simulink model "soc_swhw_fpga"  (R2021a)
settings: Solver=VariableStepAuto  StartTime=0.0  StopTime=stopTime  RelTol=1e-3  EnableMultiTasking=on
PreLoadFcn:
  | hsb.blkcb2.defineTypes;
undefined symbols (not defined in the file): a, b, Bias1, Bias2, c, frameSize, jsin, LUT_Z0, LUT_Z1, NumBits1, NumBits2, quantizationBits, sampleTime, SF, Slope1, Slope2
libraries: simulink x42, hdlsllib x24, embreciprocals x4, hwlogicconnlib x4, dsphdlxfrm x2, dsphdlmathfun x1
(part 1 of 2)
settings Model: Creator=The MathWorks, Inc.  LastModifiedBy=AliReza
settings SolverCC: AlgebraicLoopSolver=TrustRegion  PositivePriorityOrder=on
settings DataIOCC: ReturnWorkspaceOutputs=off
settings OptimizationCC: DefaultParameterBehavior=Inlined  EnhancedBackFolding=on  PassReuseOutputArgsAs=Individual arguments  MaxStackSize=64  OptimizeBlockOrder=speed  DifferentSizesBufferReuse=on  OptimizationCustomize=off  EfficientTunableParamExpr=on
settings DebuggingCC: SignalRangeChecking=warning  ParameterTunabilityLossMsg=error  SFMachineParentedDataDiag=warning  ArithmeticOperatorsInVariantConditions=warning
settings HardwareCC: ProdBitPerPointer=32  ProdBitPerSizeT=32  ProdBitPerPtrDiffT=32  ProdLargestAtomicFloat=None  ProdIntDivRoundTo=Undefined  ProdEndianess=Unspecified  ProdWordSize=32  ProdHWDeviceType=ASIC/FPGA->ASIC/FPGA  TargetBitPerPointer=64  TargetBitPerSizeT=64  TargetBitPerPtrDiffT=64  TargetLongLongMode=on  TargetIntDivRoundTo=Zero  TargetEndianess=LittleEndian  TargetWordSize=64  TargetHWDeviceType=Custom Processor->MATLAB Host Computer  ProdEqTarget=off
settings SFSimCC: SimUseLocalCustomCode=off  MATLABDynamicMemAlloc=off
settings RTWCC: SystemTargetFile=ert.tlc  TemplateMakefile=ert_default_tmf  GenerateReport=on  RTWUseLocalCustomCode=off  Toolchain=Linaro AArch32 Linux v6.3.1  IncludeHyperlinkInReport=on  LaunchReport=on  GenerateTraceInfo=on  GenerateTraceReport=on  GenerateTraceReportSl=on  GenerateTraceReportSf=on  GenerateTraceReportEml=on
settings CodeAppCC: ForceParamTrailComments=on  IgnoreCustomStorageClasses=off  OperatorAnnotations=on  SimulinkDataObjDesc=on  SFDataObjDesc=on  InsertBlockDesc=on
settings ERTTargetCC: ERTCustomFileTemplate=example_file_process.tlc

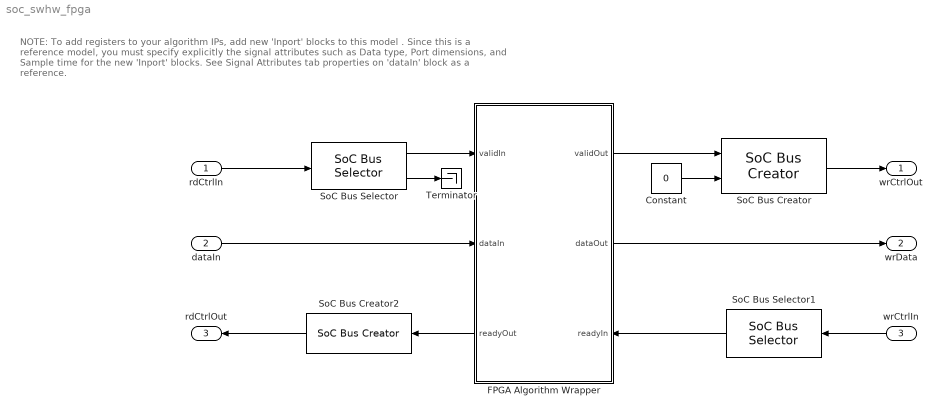
== system soc_swhw_fpga ==
  note: NOTE:
      | To add registers to your algorithm IPs, add new 'Inport' blocks to this model . Since this is a reference model, you must specify explicitly the signal attributes such as Data type, Port dimensions, and Sample time for the new 'Inport' blocks. See Signal Attributes tab properties on 'dataIn' block as a reference.
  rdCtrlIn : Inport  OutDataTypeStr=Bus: StreamM2SBusObj  SampleTime=sampleTime
  dataIn : Inport  Port=2  OutDataTypeStr=fixdt(1,32,30)  SampleTime=sampleTime
  wrCtrlIn : Inport  Port=3  OutDataTypeStr=Bus: StreamS2MBusObj  SampleTime=sampleTime
  Constant : Constant  Value=0  OutDataTypeStr=boolean  SampleTime=sampleTime
  FPGA Algorithm Wrapper : Subsystem  TreatAsAtomicUnit=on
      settings: PortSchema="{\"entries\":[{\"content\":{\"sides\":[{\"content\":{\"connectorIds\":[\"In1\",\"In2\",\"Out3\"]},\"type\":\"ConnectorPlacement.EquallySpacedRectSide\",\"uuid\":\"ebbc010d-f6ed-4988-870b-259581305fe2\"},{\"content\":{\"connectorIds\":[\"Out1\",\"Out2\",\"In3\"],\"side\":\"RIGHT\"},\"type\":\"ConnectorPlacement.EquallySpacedRectSide\",\"uuid\":\"4c5f59b6-7994-4c6f-b220-a18d8cf0d52f\"},{\"content\":{\"connectorIds\":[],\"side\":\"TOP\"},\"type\":\"ConnectorPlacement.EquallySpacedRectSide\",\"uuid\":\"7f6aff54-293a-4a30-be7c-233675f72493\"}]},\"type\":\"ConnectorPlacement.EquallySpacedConnector\",\"uuid\":\"db962109-073c-4896-87dc-fdd91b0482ef\"}],\"packageUris\":[\"http://schema.mathworks.com/mf0/Connector/R2020b\"],\"version\":\"1.0\"}"
  SoC Bus Creator : hwlogicconnlib/SoC Bus Creator  Protocol=Data stream  ctrltype=Valid
      settings: SourceProductBaseCode=HW
  SoC Bus Creator2 : hwlogicconnlib/SoC Bus Creator  Protocol=Data stream  ctrltype=Ready
      settings: SourceProductBaseCode=HW
  SoC Bus Selector : hwlogicconnlib/SoC Bus Selector  Protocol=Data stream  ctrltype=Valid
      settings: SourceProductBaseCode=HW
  SoC Bus Selector1 : hwlogicconnlib/SoC Bus Selector  Protocol=Data stream  ctrltype=Ready
      settings: SourceProductBaseCode=HW
  Terminator : Terminator
  wrCtrlOut : Outport  OutDataTypeStr=Bus: StreamM2SBusObj  SampleTime=sampleTime  InitialOutput=0
  wrData : Outport  Port=2  OutDataTypeStr=fixdt(1,32,30)  SampleTime=sampleTime  InitialOutput=0
  rdCtrlOut : Outport  Port=3  OutDataTypeStr=Bus: StreamS2MBusObj  SampleTime=sampleTime  VectorParamsAs1DForOutWhenUnconnected=off
  wires:
  FPGA Algorithm Wrapper/2(dataOut) -> wrData/1
  FPGA Algorithm Wrapper/3(readyOut) -> SoC Bus Creator2/1
  rdCtrlIn/1 -> SoC Bus Selector/1
  SoC Bus Selector/2 -> Terminator/1
  SoC Bus Selector/1 -> FPGA Algorithm Wrapper/1(validIn)
  wrCtrlIn/1 -> SoC Bus Selector1/1
  SoC Bus Selector1/1 -> FPGA Algorithm Wrapper/3(readyIn)
  SoC Bus Creator/1 -> wrCtrlOut/1
  Constant/1 -> SoC Bus Creator/2
  FPGA Algorithm Wrapper/1(validOut) -> SoC Bus Creator/1
  SoC Bus Creator2/1 -> rdCtrlOut/1
  dataIn/1 -> FPGA Algorithm Wrapper/2(dataIn)

== system soc_swhw_fpga/FPGA Algorithm Wrapper ==
  validIn : Inport
  dataIn : Inport  Port=2
  readyIn : Inport  Port=3
  Back Pressure Logic : Subsystem
      settings: PortSchema="{\"entries\":[{\"content\":{\"sides\":[{\"content\":{\"connectorIds\":[\"In1\"]},\"type\":\"ConnectorPlacement.EquallySpacedRectSide\",\"uuid\":\"912a6083-9037-4ca3-b997-83c20c2534e2\"},{\"content\":{\"connectorIds\":[\"Out1\"],\"side\":\"RIGHT\"},\"type\":\"ConnectorPlacement.EquallySpacedRectSide\",\"uuid\":\"0a4022bf-ea92-4476-83a7-d91128e221ed\"},{\"content\":{\"connectorIds\":[\"In2\",\"In3\"],\"side\":\"TOP\"},\"type\":\"ConnectorPlacement.EquallySpacedRectSide\",\"uuid\":\"948d5154-6bca-4e11-895e-98e4a1bdb5ab\"}]},\"type\":\"ConnectorPlacement.EquallySpacedConnector\",\"uuid\":\"6e974481-eff9-401c-a245-15807e59a0fd\"}],\"packageUris\":[\"http://schema.mathworks.com/mf0/Connector/R2020b\"],\"version\":\"1.0\"}"
  Enhacement Algorithm MMSE : Subsystem
  Feature Extraction : Subsystem
  Input Adapter : Subsystem
  Output Adapter : Subsystem
  validOut : Outport  InitialOutput=0
  dataOut : Outport  Port=2  InitialOutput=0
  readyOut : Outport  Port=3
  wires:
  dataIn/1 -> Input Adapter/2(dataIn)
  Output Adapter/2(dataOut) -> dataOut/1
  validIn/1 -> Back Pressure Logic/2(validIn1), Input Adapter/1(validIn)
  Output Adapter/1(validOut) -> Back Pressure Logic/3(validIn2), validOut/1
  Back Pressure Logic/1(readyOut) -> readyOut/1
  readyIn/1 -> Back Pressure Logic/1(readyIn)
  Input Adapter/3(pwrSpectrum) -> Feature Extraction/5(noisyPwrSpectrum)
  Input Adapter/2(magSpectrum) -> Enhacement Algorithm MMSE/6(noisyMagSpectrum), Feature Extraction/4(noisyMagSpectrum)
  Input Adapter/4(phaseValidOut) -> Output Adapter/3(phaseValidIn)
  Input Adapter/5(phase) -> Output Adapter/4(phaseIn)
  Enhacement Algorithm MMSE/1(enhancedMagSpectrumValid) -> Output Adapter/1(enhancedMagSpectrumValid), Feature Extraction/1(enhacedMagValidIn)
  Enhacement Algorithm MMSE/2(enhancedMagSpectrum) -> Output Adapter/2(enhancedMagSpectrum), Feature Extraction/2(enhancedMagSpectrum)
  Feature Extraction/1(aPrioriSnrValid) -> Enhacement Algorithm MMSE/1(aPrioriSnrValid)
  Feature Extraction/2(aPrioriSnr) -> Enhacement Algorithm MMSE/2(aPrioriSnr)
  Feature Extraction/3(aPosterioriSnrValid) -> Enhacement Algorithm MMSE/3(aPosterioriSnrValid)
  Input Adapter/1(SpectrumValidOut) -> Enhacement Algorithm MMSE/5(noisyMagSpectrumValid), Feature Extraction/3(noisyMagValidIn)
  Feature Extraction/4(aPosterioriSnr) -> Enhacement Algorithm MMSE/4(aPosterioriSnr)

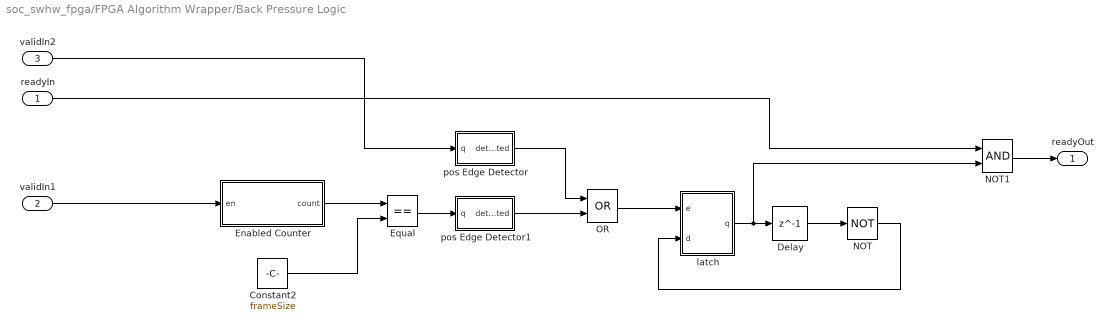
== system soc_swhw_fpga/FPGA Algorithm Wrapper/Back Pressure Logic ==
  readyIn : Inport
  validIn1 : Inport  Port=2
  validIn2 : Inport  Port=3
  Constant2 : Constant  Value=frameSize  OutDataTypeStr=fixdt(0, quantizationBits, 0)  SampleTime=-1
  Delay : Delay  DelayLength=1  InitialCondition=1
  Enabled Counter : Subsystem  TreatAsAtomicUnit=on  mask(Counter){maxCount=frameSize, sampleTime=-1}
      mask prompts: maxCount "Maximum count:"; sampleTime "Sample Time:"
  Equal : RelationalOperator  Operator===  OutDataTypeStr=boolean  RndMeth=Simplest
  NOT : Logic  Operator=NOT  AllPortsSameDT=off  OutDataTypeStr=boolean
  NOT1 : Logic  AllPortsSameDT=off  OutDataTypeStr=boolean
  OR : Logic  Operator=OR  AllPortsSameDT=off  OutDataTypeStr=boolean
  latch : Subsystem
  pos Edge Detector : Subsystem
  pos Edge Detector1 : Subsystem
  readyOut : Outport
  wires:
  Constant2/1 -> Equal/2
  Enabled Counter/1(count) -> Equal/1
  Equal/1 -> pos Edge Detector1/1(q)
  validIn1/1 -> Enabled Counter/1(en)
  Delay/1 -> NOT/1
  NOT/1 -> latch/2(d)
  pos Edge Detector1/1(detected) -> OR/2
  OR/1 -> latch/1(e)
  pos Edge Detector/1(detected) -> OR/1
  validIn2/1 -> pos Edge Detector/1(q)
  NOT1/1 -> readyOut/1
  readyIn/1 -> NOT1/1
  latch/1(q) -> NOT1/2, Delay/1

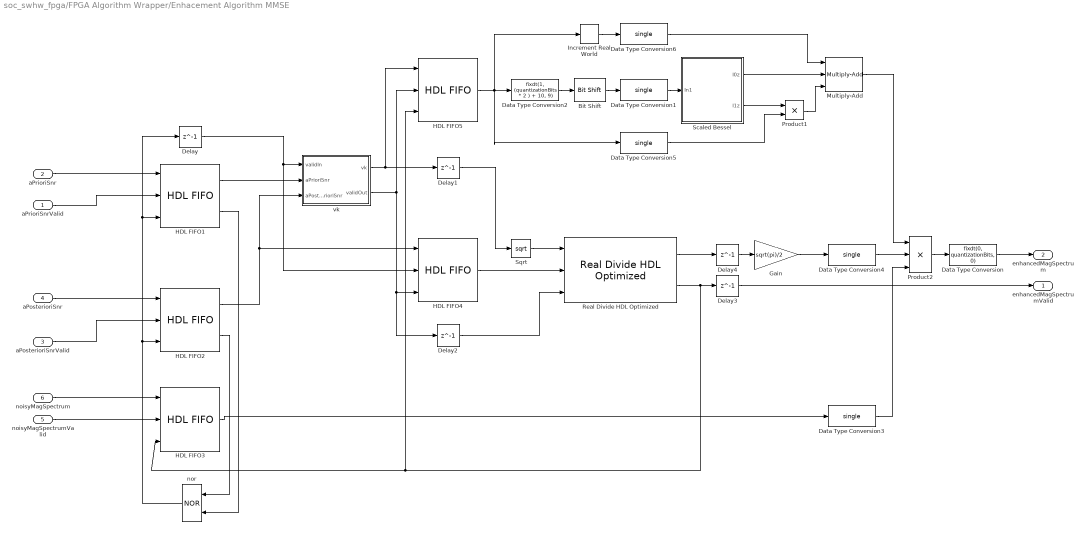
== system soc_swhw_fpga/FPGA Algorithm Wrapper/Enhacement Algorithm MMSE ==
  aPrioriSnrValid : Inport
  aPrioriSnr : Inport  Port=2
  aPosterioriSnrValid : Inport  Port=3
  aPosterioriSnr : Inport  Port=4
  noisyMagSpectrumValid : Inport  Port=5
  noisyMagSpectrum : Inport  Port=6
  Bit Shift : hdlsllib/Logic and Bit Operations/Bit Shift  mode=Shift Right Arithmetic  N=1
  Data Type Conversion : DataTypeConversion  OutDataTypeStr=fixdt(0, quantizationBits, 0)
  Data Type Conversion1 : DataTypeConversion  OutDataTypeStr=single  RndMeth=Simplest
  Data Type Conversion2 : DataTypeConversion  OutDataTypeStr=fixdt(1, (quantizationBits * 2 ) + 10, 9)
  Data Type Conversion3 : DataTypeConversion  OutDataTypeStr=single
  Data Type Conversion4 : DataTypeConversion  OutDataTypeStr=single
  Data Type Conversion5 : DataTypeConversion  OutDataTypeStr=single  RndMeth=Simplest
  Data Type Conversion6 : DataTypeConversion  OutDataTypeStr=single  RndMeth=Simplest
  Delay{,1..4} (5 alike) : Delay  DelayLength=1
  Gain : Gain  Gain=sqrt(pi)/2  ParamDataTypeStr=fixdt(0,16,16)  OutDataTypeStr=Inherit: Same as input
  HDL FIFO1 : hdlsllib/HDL RAMs/HDL FIFO  fifo_size=2^(ceil(log2(frameSize)) - 1)  mode=Classic  ratio=1  push_msg=Warning  pop_msg=Warning  show_empty=on  show_full=off  show_num=off  LabelModeActiveChoice_Mode=Classic
      settings: SourceProductBaseCode=SL
  HDL FIFO2 : hdlsllib/HDL RAMs/HDL FIFO  fifo_size=2^(ceil(log2(frameSize)) - 1)  mode=Classic  ratio=1  push_msg=Warning  pop_msg=Warning  show_empty=on  show_full=off  show_num=off  LabelModeActiveChoice_Mode=Classic
      settings: SourceProductBaseCode=SL
  HDL FIFO3 : hdlsllib/HDL RAMs/HDL FIFO  fifo_size=2^(ceil(log2(frameSize)) - 1)  mode=Classic  ratio=1  push_msg=Warning  pop_msg=Warning  show_empty=off  show_full=off  show_num=off  LabelModeActiveChoice_Mode=Classic
      settings: SourceProductBaseCode=SL
  HDL FIFO4 : hdlsllib/HDL RAMs/HDL FIFO  fifo_size=256  mode=Classic  ratio=1  push_msg=Warning  pop_msg=Warning  show_empty=off  show_full=off  show_num=off  LabelModeActiveChoice_Mode=Classic
      settings: SourceProductBaseCode=SL
  HDL FIFO5 : hdlsllib/HDL RAMs/HDL FIFO  fifo_size=256  mode=Classic  ratio=1  push_msg=Warning  pop_msg=Warning  show_empty=off  show_full=off  show_num=off  LabelModeActiveChoice_Mode=Classic
      settings: SourceProductBaseCode=SL
  Increment Real World : simulink/Additional Math & Discrete/Additional Math: Increment - Decrement/Increment Real World
      settings: SourceProductBaseCode=SL
  Multiply-Add : hdlsllib/HDL Operations/Multiply-Add  Function=c+(a.*b)  datatype=Inherit: Inherit via internal rule  RndMeth=Simplest  DoSatur=off  FMA=off
      settings: SourceProductBaseCode=SL
  Product1 : Product
  Product2 : Product  Inputs=3  RndMeth=Simplest
  Real Divide HDL Optimized : embreciprocals/Real Divide HDL Optimized  OutputType=fixdt(1, (quantizationBits * 2 ) + 17, 16)
      settings: SourceProductBaseCode=SL
  Scaled Bessel : Subsystem
  Sqrt : Sqrt  OutputSignalType=real  OutDataTypeStr=fixdt(1, (quantizationBits) + 17, 16)  SaturateOnIntegerOverflow=on
  nor : Logic  Operator=NOR  AllPortsSameDT=off  OutDataTypeStr=boolean
  vk : Subsystem
  enhancedMagSpectrumValid : Outport
  enhancedMagSpectrum : Outport  Port=2
  wires:
  noisyMagSpectrum/1 -> HDL FIFO3/1
  noisyMagSpectrumValid/1 -> HDL FIFO3/2
  aPosterioriSnrValid/1 -> HDL FIFO2/2
  aPrioriSnrValid/1 -> HDL FIFO1/2
  nor/1 -> Delay/1, HDL FIFO1/3, HDL FIFO2/3
  HDL FIFO2/2 -> nor/1
  HDL FIFO1/2 -> nor/2
  HDL FIFO1/1 -> vk/2(aPrioriSnr)
  Sqrt/1 -> Real Divide HDL Optimized/1
  Delay4/1 -> Gain/1
  HDL FIFO5/1 -> Data Type Conversion5/1, Increment Real World/1, Data Type Conversion2/1
  Data Type Conversion1/1 -> Scaled Bessel/1(In1)
  Scaled Bessel/1(I0z) -> Multiply-Add/2
  Increment Real World/1 -> Data Type Conversion6/1
  Scaled Bessel/2(I1z) -> Product1/1
  Product1/1 -> Multiply-Add/3
  Gain/1 -> Data Type Conversion4/1
  HDL FIFO3/1 -> Data Type Conversion3/1
  Product2/1 -> Data Type Conversion/1
  Delay/1 -> HDL FIFO4/2, vk/1(validIn)
  Data Type Conversion/1 -> enhancedMagSpectrum/1
  HDL FIFO4/1 -> Real Divide HDL Optimized/2
  vk/2(validOut) -> Delay2/1, HDL FIFO4/3, HDL FIFO5/2
  Delay2/1 -> Real Divide HDL Optimized/3
  Delay1/1 -> Sqrt/1
  vk/1(vk) -> Delay1/1, HDL FIFO5/1
  Real Divide HDL Optimized/2 -> Delay3/1, HDL FIFO3/3, HDL FIFO5/3
  Delay3/1 -> enhancedMagSpectrumValid/1
  Real Divide HDL Optimized/1 -> Delay4/1
  Data Type Conversion3/1 -> Product2/3
  aPosterioriSnr/1 -> HDL FIFO2/1
  aPrioriSnr/1 -> HDL FIFO1/1
  HDL FIFO2/1 -> HDL FIFO4/1, vk/3(aPosterioriSnr)
  Bit Shift/1 -> Data Type Conversion1/1
  Data Type Conversion2/1 -> Bit Shift/1
  Data Type Conversion4/1 -> Product2/2
  Multiply-Add/1 -> Product2/1
  Data Type Conversion5/1 -> Product1/2
  Data Type Conversion6/1 -> Multiply-Add/1

== system soc_swhw_fpga/FPGA Algorithm Wrapper/Feature Extraction ==
  enhacedMagValidIn : Inport
  enhancedMagSpectrum : Inport  Port=2
  noisyMagValidIn : Inport  Port=3
  noisyMagSpectrum : Inport  Port=4
  noisyPwrSpectrum : Inport  Port=5
  VAD : Subsystem  Commented=on
  aPosterioriSNR : Subsystem
  aPrioriSNR : Subsystem
  aPrioriSnrValid : Outport
  aPrioriSnr : Outport  Port=2
  aPosterioriSnrValid : Outport  Port=3
  aPosterioriSnr : Outport  Port=4
  wires:
  aPrioriSNR/1(validOut) -> aPrioriSnrValid/1
  aPrioriSNR/2(aPrioriSnr) -> aPrioriSnr/1
  aPosterioriSNR/3(noisePwrSpectrum) -> aPrioriSNR/5(noisePwrSpectrum)
  enhacedMagValidIn/1 -> aPrioriSNR/1(MagValidIn)
  noisyPwrSpectrum/1 -> aPosterioriSNR/3(pwrSpectrum)
  noisyMagSpectrum/1 -> aPosterioriSNR/2(magSpectrum)
  enhancedMagSpectrum/1 -> aPrioriSNR/2(enhancedMagSpectrum)
  aPosterioriSNR/2(aPosterioriSNR) -> aPrioriSNR/3(aPosterioriSNR), aPosterioriSnr/1
  aPosterioriSNR/1(validOut) -> aPrioriSNR/4(SnrValidIn), aPosterioriSnrValid/1
  noisyMagValidIn/1 -> aPosterioriSNR/1(validIn)

== system soc_swhw_fpga/FPGA Algorithm Wrapper/Input Adapter ==
  validIn : Inport
  dataIn : Inport  Port=2
  FFT : Subsystem
  Hamming Window : Subsystem  TreatAsAtomicUnit=on
  Quantize : Subsystem  TreatAsAtomicUnit=on
  Single-Sided Spectrum : Subsystem
  Zero Pad : Subsystem
  SpectrumValidOut : Outport
  magSpectrum : Outport  Port=2
  pwrSpectrum : Outport  Port=3
  phaseValidOut : Outport  Port=4
  phase : Outport  Port=5
  wires:
  dataIn/1 -> Quantize/2(dataIn)
  Quantize/1(validOut) -> Hamming Window/1(validIn)
  Quantize/2(dataOut) -> Hamming Window/2(dataIn)
  Hamming Window/1(validOut) -> Zero Pad/1(validIn)
  Hamming Window/2(dataOut) -> Zero Pad/2(dataIn)
  Zero Pad/1(validOut) -> FFT/1(validIn)
  Zero Pad/2(dataOut) -> FFT/2(dataIn)
  validIn/1 -> Quantize/1(validIn)
  FFT/1(validOut) -> Single-Sided Spectrum/1(validIn)
  FFT/2(dataOut) -> Single-Sided Spectrum/2(dataIn)
  Single-Sided Spectrum/1(SpectrumValidOut) -> SpectrumValidOut/1
  Single-Sided Spectrum/2(magSpectrum) -> magSpectrum/1
  Single-Sided Spectrum/3(pwrSpectrum) -> pwrSpectrum/1
  Single-Sided Spectrum/4(phaseValidOut) -> phaseValidOut/1
  Single-Sided Spectrum/5(phase) -> phase/1

== system soc_swhw_fpga/FPGA Algorithm Wrapper/Output Adapter ==
  enhancedMagSpectrumValid : Inport
  enhancedMagSpectrum : Inport  Port=2
  phaseValidIn : Inport  Port=3
  phaseIn : Inport  Port=4
  De-Quantize : Subsystem  TreatAsAtomicUnit=on
  IFFT : Subsystem
  Magnitude and Phase to Complex : Subsystem
  Spectrum Mirror : Subsystem
  Zero Chop : Subsystem
  validOut : Outport
  dataOut : Outport  Port=2
  wires:
  IFFT/2(dataOut) -> Zero Chop/2(dataIn)
  IFFT/1(validOut) -> Zero Chop/1(validIn)
  De-Quantize/1(validOut) -> validOut/1
  De-Quantize/2(dataOut) -> dataOut/1
  enhancedMagSpectrum/1 -> Spectrum Mirror/2(dataIn)
  enhancedMagSpectrumValid/1 -> Spectrum Mirror/1(validIn)
  Zero Chop/1(validOut) -> De-Quantize/1(validIn)
  Zero Chop/2(dataOut) -> De-Quantize/2(dataIn)
  Spectrum Mirror/1(validOut) -> Magnitude and Phase to Complex/1(magnitudeValidIn)
  Spectrum Mirror/2(dataOut) -> Magnitude and Phase to Complex/2(magnitudeIn)
  Magnitude and Phase to Complex/1(validOut) -> IFFT/1(validIn)
  Magnitude and Phase to Complex/2(dataOut) -> IFFT/2(dataIn)
  phaseValidIn/1 -> Magnitude and Phase to Complex/3(phaseValidIn)
  phaseIn/1 -> Magnitude and Phase to Complex/4(phaseIn)

== system soc_swhw_fpga/FPGA Algorithm Wrapper/Back Pressure Logic/Enabled Counter ==
  en : Inport
  Add : Sum  AccumDataTypeStr=uint(floor(log2(maxCount))+1)  OutDataTypeStr=uint(floor(log2(maxCount))+1)  RndMeth=Simplest
  Compare To Constant : simulink/Logic and Bit Operations/Compare To Constant  relop===  const=maxCount  OutDataTypeStr=boolean
  Constant : Constant  OutDataTypeStr=uint(floor(log2(maxCount))+1)  SampleTime=-1
  Constant1 : Constant  Value=0  OutDataTypeStr=uint(floor(log2(maxCount))+1)  SampleTime=-1
  Delay One Step : Delay  DelayLength=1  InitialCondition=0
  Delay One Step1 : Delay  DelayLength=1  InitialCondition=0
  Multiport Switch : MultiPortSwitch  DataPortOrder=Zero-based contiguous  Inputs=2  zeroidx=on
  Multiport Switch1 : MultiPortSwitch  DataPortOrder=Zero-based contiguous  Inputs=2  zeroidx=on
  Multiport Switch2 : MultiPortSwitch  DataPortOrder=Zero-based contiguous  Inputs=2  zeroidx=on
  count : Outport
  wires:
  Constant/1 -> Add/1
  en/1 -> Multiport Switch1/1, Multiport Switch/1
  Add/1 -> Multiport Switch/3
  Multiport Switch/1 -> Multiport Switch2/2, Multiport Switch1/3, Compare To Constant/1
  Delay One Step/1 -> Multiport Switch/2, Add/2
  Compare To Constant/1 -> Multiport Switch2/1
  Delay One Step1/1 -> Multiport Switch1/2
  Multiport Switch1/1 -> count/1, Delay One Step1/1
  Multiport Switch2/1 -> Delay One Step/1
  Constant1/1 -> Multiport Switch2/3

== system soc_swhw_fpga/FPGA Algorithm Wrapper/Back Pressure Logic/latch ==
  e : Inport
  d : Inport  Port=2
  Delay : Delay  DelayLength=1  InitialCondition=1
  Switch : Switch  Criteria=u2 ~= 0  RndMeth=Simplest
  q : Outport
  wires:
  Switch/1 -> q/1, Delay/1
  Delay/1 -> Switch/3
  e/1 -> Switch/2
  d/1 -> Switch/1

== system soc_swhw_fpga/FPGA Algorithm Wrapper/Back Pressure Logic/pos Edge Detector ==
  q : Inport
  AND : Logic  AllPortsSameDT=off  OutDataTypeStr=boolean
  Delay1 : Delay  DelayLength=1
  XOR : Logic  Operator=XOR  AllPortsSameDT=off  OutDataTypeStr=boolean
  detected : Outport
  wires:
  XOR/1 -> AND/1
  Delay1/1 -> XOR/2
  q/1 -> XOR/1, AND/2, Delay1/1
  AND/1 -> detected/1

== system soc_swhw_fpga/FPGA Algorithm Wrapper/Back Pressure Logic/pos Edge Detector1 ==
  q : Inport
  AND : Logic  AllPortsSameDT=off  OutDataTypeStr=boolean
  Delay1 : Delay  DelayLength=1
  XOR : Logic  Operator=XOR  AllPortsSameDT=off  OutDataTypeStr=boolean
  detected : Outport
  wires:
  XOR/1 -> AND/1
  Delay1/1 -> XOR/2
  q/1 -> XOR/1, AND/2, Delay1/1
  AND/1 -> detected/1

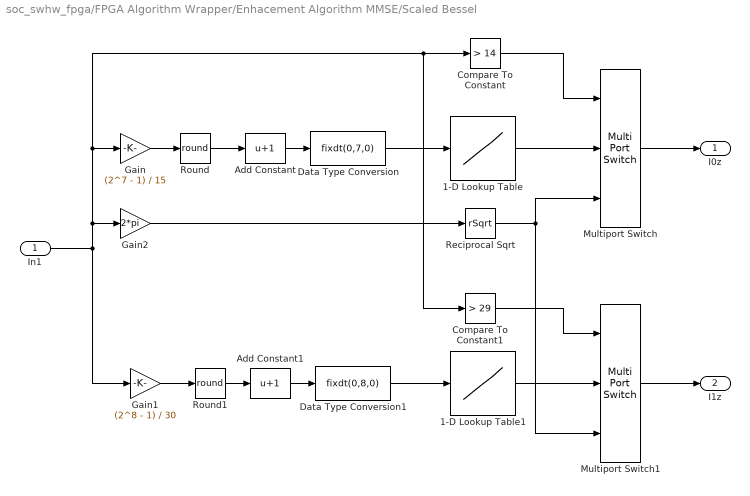
== system soc_swhw_fpga/FPGA Algorithm Wrapper/Enhacement Algorithm MMSE/Scaled Bessel ==
  In1 : Inport
  1-D Lookup Table : Lookup_n-D  NumberOfTableDimensions=1  BreakpointsForDimension1=[0 : 127]  BreakpointsForDimension1FirstPoint=0  IndexSearchMethod=Evenly spaced points  Table=LUT_Z0  TableDataTypeStr=single  InterpMethod=Flat  RemoveProtectionInput=on  InternalRulePriority=Speed  OutDataTypeStr=single  RndMeth=Simplest
  1-D Lookup Table1 : Lookup_n-D  NumberOfTableDimensions=1  BreakpointsForDimension1=[0 : 255]  BreakpointsForDimension1FirstPoint=0  IndexSearchMethod=Evenly spaced points  Table=LUT_Z1  TableDataTypeStr=single  InterpMethod=Flat  RemoveProtectionInput=on  InternalRulePriority=Speed  OutDataTypeStr=single  RndMeth=Zero
  Add Constant : Bias  Bias=1
  Add Constant1 : Bias  Bias=1
  Compare To Constant : simulink/Logic and Bit Operations/Compare To Constant  relop=>  const=14  OutDataTypeStr=boolean
  Compare To Constant1 : simulink/Logic and Bit Operations/Compare To Constant  relop=>  const=29  OutDataTypeStr=boolean
  Data Type Conversion : DataTypeConversion  OutDataTypeStr=fixdt(0,7,0)  RndMeth=Zero
  Data Type Conversion1 : DataTypeConversion  OutDataTypeStr=fixdt(0,8,0)
  Gain : Gain  Gain=(2^7 - 1) / 15
  Gain1 : Gain  Gain=(2^8 - 1) / 30
  Gain2 : Gain  Gain=2*pi
  Multiport Switch : MultiPortSwitch  DataPortOrder=Zero-based contiguous  Inputs=2  zeroidx=on
  Multiport Switch1 : MultiPortSwitch  DataPortOrder=Zero-based contiguous  Inputs=2  zeroidx=on
  Reciprocal Sqrt : Sqrt  Operator=rSqrt  SaturateOnIntegerOverflow=on
  Round : Rounding  Operator=round
  Round1 : Rounding  Operator=round
  I0z : Outport
  I1z : Outport  Port=2
  wires:
  Multiport Switch/1 -> I0z/1
  Multiport Switch1/1 -> I1z/1
  Compare To Constant/1 -> Multiport Switch/1
  Reciprocal Sqrt/1 -> Multiport Switch/3, Multiport Switch1/3
  Compare To Constant1/1 -> Multiport Switch1/1
  Add Constant/1 -> Data Type Conversion/1
  Add Constant1/1 -> Data Type Conversion1/1
  Round/1 -> Add Constant/1
  Round1/1 -> Add Constant1/1
  Gain/1 -> Round/1
  Gain1/1 -> Round1/1
  In1/1 -> Gain/1, Compare To Constant1/1, Compare To Constant/1, Gain2/1, Gain1/1
  Gain2/1 -> Reciprocal Sqrt/1
  Data Type Conversion/1 -> 1-D Lookup Table/1
  Data Type Conversion1/1 -> 1-D Lookup Table1/1
  1-D Lookup Table/1 -> Multiport Switch/2
  1-D Lookup Table1/1 -> Multiport Switch1/2

== system soc_swhw_fpga/FPGA Algorithm Wrapper/Enhacement Algorithm MMSE/vk ==
  validIn : Inport
  aPrioriSnr : Inport  Port=2
  aPosterioriSnr : Inport  Port=3
  Delay : Delay  DelayLength=1
  Delay1 : Delay  DelayLength=1
  HDL FIFO4 : hdlsllib/HDL RAMs/HDL FIFO  fifo_size=256  mode=Classic  ratio=1  push_msg=Warning  pop_msg=Warning  show_empty=off  show_full=off  show_num=off  LabelModeActiveChoice_Mode=Classic
      settings: SourceProductBaseCode=SL
  Increment Real World : simulink/Additional Math & Discrete/Additional Math: Increment - Decrement/Increment Real World
      settings: SourceProductBaseCode=SL
  Product : Product  OutDataTypeStr=Inherit: Same as first input
  Real Divide HDL Optimized : embreciprocals/Real Divide HDL Optimized  OutputType=fixdt(1, (quantizationBits * 2 ) + 9, 8)
      settings: SourceProductBaseCode=SL
  vk : Outport
  validOut : Outport  Port=2
  wires:
  Real Divide HDL Optimized/1 -> Delay/1
  aPosterioriSnr/1 -> HDL FIFO4/1
  aPrioriSnr/1 -> Increment Real World/1, Real Divide HDL Optimized/1
  Real Divide HDL Optimized/2 -> HDL FIFO4/3, Delay1/1
  validIn/1 -> HDL FIFO4/2, Real Divide HDL Optimized/3
  Increment Real World/1 -> Real Divide HDL Optimized/2
  HDL FIFO4/1 -> Product/2
  Delay/1 -> Product/1
  Delay1/1 -> validOut/1
  Product/1 -> vk/1

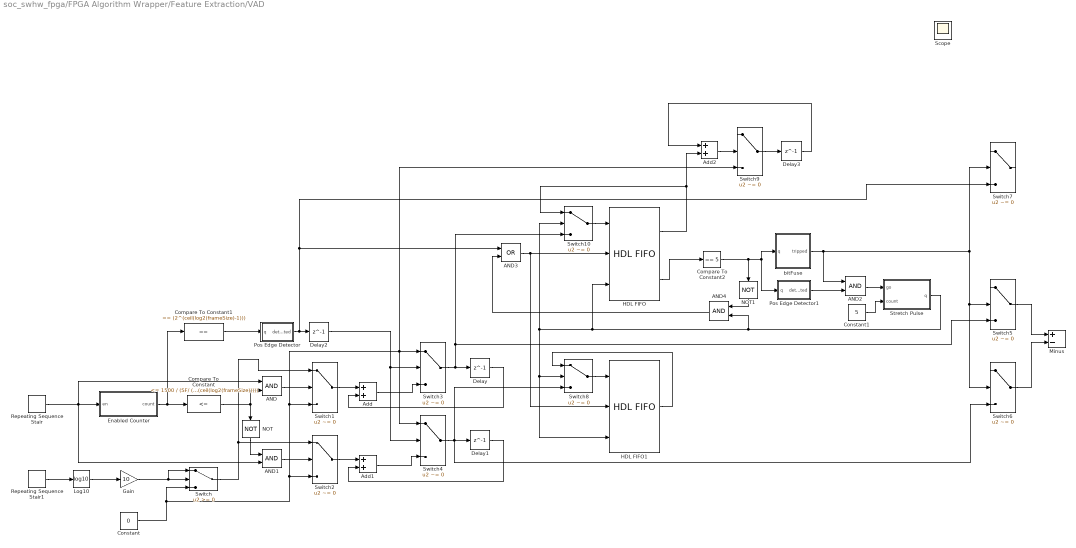
== system soc_swhw_fpga/FPGA Algorithm Wrapper/Feature Extraction/VAD ==
  AND{,1..2,4} (4 alike) : Logic  AllPortsSameDT=off  OutDataTypeStr=boolean
  AND3 : Logic  Operator=OR  AllPortsSameDT=off  OutDataTypeStr=boolean
  Add : Sum
  Add1 : Sum
  Add2 : Sum
  Compare To Constant : simulink/Logic and Bit Operations/Compare To Constant  relop=<=  const=1500 / (SF/ (2^(ceil(log2(frameSize)))))  OutDataTypeStr=boolean
  Compare To Constant1 : simulink/Logic and Bit Operations/Compare To Constant  relop===  const=(2^(ceil(log2(frameSize)-1)))  OutDataTypeStr=boolean  ZeroCross=off
  Compare To Constant2 : simulink/Logic and Bit Operations/Compare To Constant  relop===  const=5  OutDataTypeStr=boolean
  Constant : Constant  Value=0
  Constant1 : Constant  Value=5
  Delay{,1..3} (4 alike) : Delay  DelayLength=1
  Enabled Counter : Subsystem  TreatAsAtomicUnit=on  mask(Counter){maxCount=256, sampleTime=-1}
      mask prompts: maxCount "Maximum count:"; sampleTime "Sample Time:"
  Gain : Gain  Gain=10
  HDL FIFO : hdlsllib/HDL RAMs/HDL FIFO  fifo_size=5  mode=Classic  ratio=1  push_msg=Error  pop_msg=Error  show_empty=off  show_full=off  show_num=on  LabelModeActiveChoice_Mode=Classic
      settings: SourceProductBaseCode=SL
  HDL FIFO1 : hdlsllib/HDL RAMs/HDL FIFO  fifo_size=5  mode=Classic  ratio=1  push_msg=Error  pop_msg=Error  show_empty=off  show_full=off  show_num=off  LabelModeActiveChoice_Mode=Classic
      settings: SourceProductBaseCode=SL
  Log10 : Math  Operator=log10  SaturateOnIntegerOverflow=on
  Minus : Sum  Inputs=+-
  NOT : Logic  Operator=NOT  IconShape=distinctive  AllPortsSameDT=off  OutDataTypeStr=boolean
  NOT1 : Logic  Operator=NOT  IconShape=distinctive  AllPortsSameDT=off  OutDataTypeStr=boolean
  Pos Edge Detector : Subsystem
  Pos Edge Detector1 : Subsystem
  Repeating Sequence Stair : simulink/Sources/Repeating Sequence Stair  OutValues=[0 0 0 0 0 1 0 1 0 1 0 1 0 1 0 0 0 0 1 1 1 1 1 1 0 0 0 0 0 0 0 0 0 0]  tsamp=1  OutMin=[]  OutMax=[]  OutDataTypeStr=fixdt('boolean')  OutputDataTypeScalingMode=Specify via dialog  OutDataType=fixdt('boolean')  ConRadixGroup=Best Precision: Vector-wise  OutScaling=[]
  Repeating Sequence Stair1 : simulink/Sources/Repeating Sequence Stair  OutValues=[0 0 0 0 0 1 0 1 0 1 0 1 0 1 0 0 0 0 1 1 1 1 1 1 0 0 0 0 0 0 0 0 0 0]  tsamp=1  OutMin=[]  OutMax=[]  OutDataTypeStr=fixdt('boolean')  OutputDataTypeScalingMode=Specify via dialog  OutDataType=fixdt('boolean')  ConRadixGroup=Best Precision: Vector-wise  OutScaling=[]
  Scope : Scope  NumInputPorts=2
  Stretch Pulse : Subsystem
  Switch : Switch
  Switch{1..10} (10 alike) : Switch  Criteria=u2 ~= 0
  bitFuse : Subsystem
  wires:
  HDL FIFO/1 -> Switch10/1, Add2/2
  HDL FIFO1/1 -> Switch8/1
  Switch10/1 -> HDL FIFO/1
  AND4/1 -> AND3/2
  Switch8/1 -> HDL FIFO1/1
  AND3/1 -> HDL FIFO1/2, HDL FIFO/2
  Constant1/1 -> Stretch Pulse/2(count)
  Delay3/1 -> Add2/1
  Switch9/1 -> Delay3/1
  Stretch Pulse/1(q) -> Switch10/2, HDL FIFO1/3, Switch8/2, HDL FIFO/3, AND4/2
  Repeating Sequence Stair1/1 -> Log10/1
  Switch1/1 -> Add/1
  bitFuse/1(tripped) -> AND2/1, Switch7/2, Switch6/2, Switch5/2
  Repeating Sequence Stair/1 -> AND/1, AND1/2, Enabled Counter/1(en)
  Delay2/1 -> Switch4/2, Switch3/2
  HDL FIFO/2 -> Compare To Constant2/1
  Gain/1 -> Switch/1, Switch/2
  Enabled Counter/1(count) -> Compare To Constant1/1, Compare To Constant/1
  Switch4/1 -> Switch8/3, Switch6/3, Delay1/1
  Switch/1 -> Switch2/1, Switch1/1
  Switch2/1 -> Add1/1
  AND/1 -> Switch1/2
  Delay/1 -> Add/2
  Constant/1 -> Switch2/3, Switch1/3, Switch4/1, Switch9/3, Switch3/1, Switch/3
  AND1/1 -> Switch2/2
  Log10/1 -> Gain/1
  Pos Edge Detector1/1(detected) -> AND2/2
  Switch5/1 -> Minus/1
  Delay1/1 -> Add1/2
  Compare To Constant/1 -> AND/2, NOT/1
  Pos Edge Detector/1(detected) -> Switch7/3, AND3/1, Delay2/1
  Add1/1 -> Switch4/3
  Switch6/1 -> Minus/2
  Add/1 -> Switch3/3
  Compare To Constant2/1 -> NOT1/1, Pos Edge Detector1/1(q), bitFuse/1(q)
  NOT/1 -> AND1/1
  AND2/1 -> Stretch Pulse/1(go)
  Compare To Constant1/1 -> Pos Edge Detector/1(q)
  NOT1/1 -> AND4/1
  Add2/1 -> Switch9/2
  Switch3/1 -> Switch10/3, Switch5/3, Delay/1

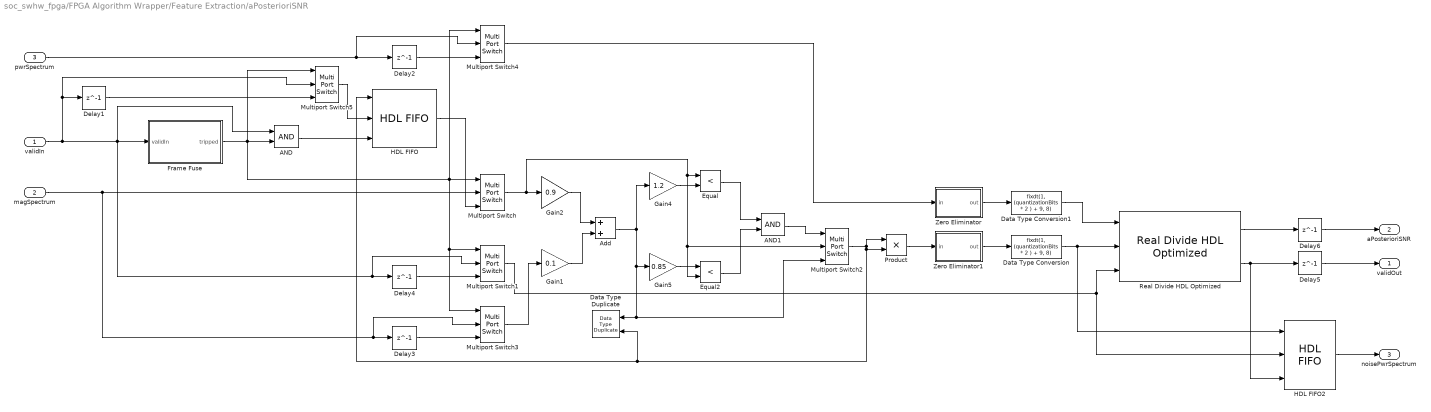
== system soc_swhw_fpga/FPGA Algorithm Wrapper/Feature Extraction/aPosterioriSNR ==
  validIn : Inport
  magSpectrum : Inport  Port=2
  pwrSpectrum : Inport  Port=3
  AND : Logic  AllPortsSameDT=off  OutDataTypeStr=boolean
  AND1 : Logic  AllPortsSameDT=off  OutDataTypeStr=boolean
  Add : Sum  OutDataTypeStr=Inherit: Same as first input
  Data Type Duplicate : DataTypeDuplicate
  Data Type Conversion : DataTypeConversion  OutDataTypeStr=fixdt(1, (quantizationBits * 2 ) + 9, 8)  SaturateOnIntegerOverflow=on  RndMeth=Zero
  Data Type Conversion1 : DataTypeConversion  OutDataTypeStr=fixdt(1, (quantizationBits * 2 ) + 9, 8)  SaturateOnIntegerOverflow=on  RndMeth=Zero
  Delay{1..6} (6 alike) : Delay  DelayLength=1
  Equal : RelationalOperator  Operator=<  OutDataTypeStr=boolean  RndMeth=Simplest
  Equal2 : RelationalOperator  Operator=<  OutDataTypeStr=boolean  RndMeth=Simplest
  Frame Fuse : Subsystem
  Gain1 : Gain  Gain=0.1  ParamDataTypeStr=fixdt(0,8,8)  RndMeth=Zero  OutDataTypeStr=Inherit: Same as input
  Gain2 : Gain  Gain=0.9  ParamDataTypeStr=fixdt(0,8,8)  RndMeth=Zero  OutDataTypeStr=Inherit: Same as input
  Gain4 : Gain  Gain=1.2  ParamDataTypeStr=fixdt(0,8,7)  OutDataTypeStr=fixdt(0, quantizationBits + 1, 0)  RndMeth=Zero
  Gain5 : Gain  Gain=0.85  ParamDataTypeStr=fixdt(0,8,8)  RndMeth=Zero  OutDataTypeStr=Inherit: Same as input
  HDL FIFO : hdlsllib/HDL RAMs/HDL FIFO  fifo_size=2^(ceil(log2(frameSize)) - 1)  mode=Classic  ratio=1  push_msg=Warning  pop_msg=Warning  show_empty=off  show_full=off  show_num=off  LabelModeActiveChoice_Mode=Classic
      settings: SourceProductBaseCode=SL
  HDL FIFO2 : hdlsllib/HDL RAMs/HDL FIFO  fifo_size=2^(ceil(log2(frameSize)) - 1)  mode=Classic  ratio=1  push_msg=Warning  pop_msg=Warning  show_empty=off  show_full=off  show_num=off  LabelModeActiveChoice_Mode=Classic
      settings: SourceProductBaseCode=SL
  Multiport Switch{,1..5} (6 alike) : MultiPortSwitch  DataPortOrder=Zero-based contiguous  Inputs=2  zeroidx=on
  Product : Product
  Real Divide HDL Optimized : embreciprocals/Real Divide HDL Optimized  OutputType=fixdt(1, (quantizationBits * 2 ) + 9, 8)
      settings: SourceProductBaseCode=SL
  Zero Eliminator : Subsystem
  Zero Eliminator1 : Subsystem
  validOut : Outport
  aPosterioriSNR : Outport  Port=2
  noisePwrSpectrum : Outport  Port=3
  wires:
  Frame Fuse/1(tripped) -> AND/2, Multiport Switch5/1, Multiport Switch/1, Multiport Switch1/1, Multiport Switch3/1, Multiport Switch4/1
  AND/1 -> HDL FIFO/3
  validIn/1 -> Multiport Switch5/2, Delay1/1, Multiport Switch1/2, Delay4/1, AND/1, Frame Fuse/1(validIn)
  HDL FIFO/1 -> Multiport Switch/3
  magSpectrum/1 -> Multiport Switch3/2, Delay3/1, Multiport Switch/2
  Gain2/1 -> Add/1
  Gain1/1 -> Add/2
  Multiport Switch/1 -> Multiport Switch2/2, Equal2/2, Equal/1, Gain2/1
  Add/1 -> Gain4/1, Data Type Duplicate/1, Multiport Switch2/3, Gain5/1
  Gain4/1 -> Equal/2
  Gain5/1 -> Equal2/1
  Equal/1 -> AND1/1
  Equal2/1 -> AND1/2
  AND1/1 -> Multiport Switch2/1
  Product/1 -> Zero Eliminator1/1(in)
  Data Type Conversion1/1 -> Real Divide HDL Optimized/1
  Real Divide HDL Optimized/2 -> Delay5/1, HDL FIFO2/3
  Delay3/1 -> Multiport Switch3/3
  Delay4/1 -> Multiport Switch1/3
  Multiport Switch3/1 -> Gain1/1
  pwrSpectrum/1 -> Delay2/1, Multiport Switch4/2
  Delay2/1 -> Multiport Switch4/3
  Multiport Switch4/1 -> Zero Eliminator/1(in)
  Multiport Switch2/1 -> HDL FIFO/1, Data Type Duplicate/2, Product/2, Product/1
  Multiport Switch5/1 -> HDL FIFO/2
  Delay1/1 -> Multiport Switch5/3
  Zero Eliminator/1(out) -> Data Type Conversion1/1
  Real Divide HDL Optimized/1 -> Delay6/1
  Zero Eliminator1/1(out) -> Data Type Conversion/1
  Delay5/1 -> validOut/1
  Delay6/1 -> aPosterioriSNR/1
  HDL FIFO2/1 -> noisePwrSpectrum/1
  Data Type Conversion/1 -> HDL FIFO2/1, Real Divide HDL Optimized/2
  Multiport Switch1/1 -> Real Divide HDL Optimized/3, HDL FIFO2/2

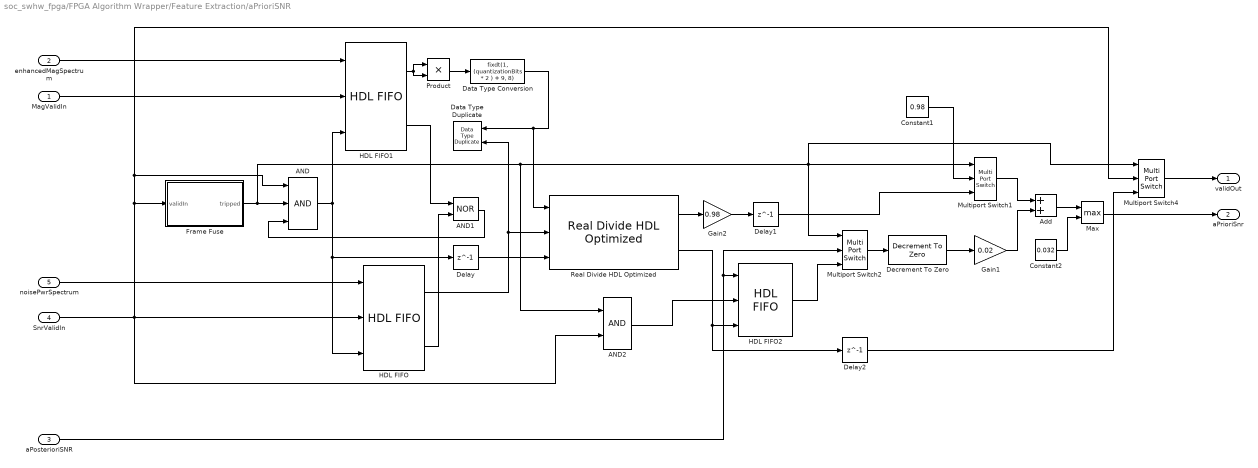
== system soc_swhw_fpga/FPGA Algorithm Wrapper/Feature Extraction/aPrioriSNR ==
  MagValidIn : Inport
  enhancedMagSpectrum : Inport  Port=2
  aPosterioriSNR : Inport  Port=3
  SnrValidIn : Inport  Port=4
  noisePwrSpectrum : Inport  Port=5
  AND : Logic  Inputs=3  AllPortsSameDT=off  OutDataTypeStr=boolean
  AND1 : Logic  Operator=NOR  AllPortsSameDT=off  OutDataTypeStr=boolean
  AND2 : Logic  AllPortsSameDT=off  OutDataTypeStr=boolean
  Add : Sum  OutDataTypeStr=Inherit: Same as first input
  Constant1 : Constant  Value=0.98  OutDataTypeStr=fixdt(0, 8, 8)  SampleTime=sampleTime
  Constant2 : Constant  Value=0.032  OutDataTypeStr=fixdt(0, 8, 8)  SampleTime=sampleTime
  Data Type Duplicate : DataTypeDuplicate
  Data Type Conversion : DataTypeConversion  OutDataTypeStr=fixdt(1, (quantizationBits * 2 ) + 9, 8)
  Decrement To Zero : simulink/Additional Math & Discrete/Additional Math: Increment - Decrement/Decrement To Zero
      settings: SourceProductBaseCode=SL
  Delay : Delay  DelayLength=1
  Delay1 : Delay  DelayLength=1
  Delay2 : Delay  DelayLength=1
  Frame Fuse : Subsystem
  Gain1 : Gain  Gain=0.02  ParamDataTypeStr=fixdt(0, 8, 8)  RndMeth=Zero  OutDataTypeStr=Inherit: Same as input
  Gain2 : Gain  Gain=0.98  ParamDataTypeStr=fixdt(0, 8, 8)  RndMeth=Zero  OutDataTypeStr=Inherit: Same as input
  HDL FIFO : hdlsllib/HDL RAMs/HDL FIFO  fifo_size=2^(ceil(log2(frameSize)) - 1)  mode=Classic  ratio=1  push_msg=Warning  pop_msg=Warning  show_empty=on  show_full=off  show_num=off  LabelModeActiveChoice_Mode=Classic
      settings: SourceProductBaseCode=SL
  HDL FIFO1 : hdlsllib/HDL RAMs/HDL FIFO  fifo_size=2^(ceil(log2(frameSize)) - 1)  mode=Classic  ratio=1  push_msg=Warning  pop_msg=Warning  show_empty=on  show_full=off  show_num=off  LabelModeActiveChoice_Mode=Classic
      settings: SourceProductBaseCode=SL
  HDL FIFO2 : hdlsllib/HDL RAMs/HDL FIFO  fifo_size=2^(ceil(log2(frameSize)) - 1)  mode=Classic  ratio=1  push_msg=Warning  pop_msg=Warning  show_empty=off  show_full=off  show_num=off  LabelModeActiveChoice_Mode=Classic
      settings: SourceProductBaseCode=SL
  Max : MinMax  Function=max  Inputs=2
  Multiport Switch1 : MultiPortSwitch  DataPortOrder=Zero-based contiguous  Inputs=2  zeroidx=on
  Multiport Switch2 : MultiPortSwitch  DataPortOrder=Zero-based contiguous  Inputs=2  zeroidx=on
  Multiport Switch4 : MultiPortSwitch  DataPortOrder=Zero-based contiguous  Inputs=2  zeroidx=on
  Product : Product
  Real Divide HDL Optimized : embreciprocals/Real Divide HDL Optimized  OutputType=fixdt(1, (quantizationBits * 2 ) + 9, 8)
      settings: SourceProductBaseCode=SL
  validOut : Outport
  aPrioriSnr : Outport  Port=2
  wires:
  MagValidIn/1 -> HDL FIFO1/2
  enhancedMagSpectrum/1 -> HDL FIFO1/1
  SnrValidIn/1 -> AND2/2, AND/1, Multiport Switch4/2, Frame Fuse/1(validIn), HDL FIFO/2
  HDL FIFO1/1 -> Product/1, Product/2
  noisePwrSpectrum/1 -> HDL FIFO/1
  Frame Fuse/1(tripped) -> AND/2, AND2/1, Multiport Switch2/1, Multiport Switch1/1, Multiport Switch4/1
  HDL FIFO1/2 -> AND1/1
  HDL FIFO/2 -> AND1/2
  AND1/1 -> AND/3
  AND/1 -> HDL FIFO/3, Delay/1, HDL FIFO1/3
  Data Type Conversion/1 -> Data Type Duplicate/1, Real Divide HDL Optimized/1
  HDL FIFO/1 -> Data Type Duplicate/2, Real Divide HDL Optimized/2
  Delay/1 -> Real Divide HDL Optimized/3
  Real Divide HDL Optimized/1 -> Gain2/1
  Gain2/1 -> Delay1/1
  Multiport Switch1/1 -> Add/1
  Gain1/1 -> Add/2
  Decrement To Zero/1 -> Gain1/1
  Add/1 -> Max/1
  Constant2/1 -> Max/2
  Multiport Switch4/1 -> validOut/1
  Max/1 -> aPrioriSnr/1
  Real Divide HDL Optimized/2 -> Delay2/1, HDL FIFO2/3
  Multiport Switch2/1 -> Decrement To Zero/1
  aPosterioriSNR/1 -> Multiport Switch2/2, HDL FIFO2/1
  AND2/1 -> HDL FIFO2/2
  HDL FIFO2/1 -> Multiport Switch2/3
  Delay1/1 -> Multiport Switch1/3
  Delay2/1 -> Multiport Switch4/3
  Constant1/1 -> Multiport Switch1/2
  Product/1 -> Data Type Conversion/1

== system soc_swhw_fpga/FPGA Algorithm Wrapper/Input Adapter/FFT ==
  validIn : Inport
  dataIn : Inport  Port=2
  FFT HDL Optimized : dsphdlxfrm/FFT HDL Optimized  FFTLength=(2 ^ (floor(log2(frameSize)) + 1))  Architecture=Burst Radix 2  ComplexMultiplication=Use 3 multipliers and 5 adders  BitReversedOutput=off  BitReversedInput=off  Normalize=on  SimulateUsing=Code generation  RoundingMethod=Zero  ResetInputPort=off  StartOutputPort=off  EndOutputPort=off
      settings: SourceProductBaseCode=DS
  Terminator : Terminator
  validOut : Outport
  dataOut : Outport  Port=2
  wires:
  validIn/1 -> FFT HDL Optimized/2
  FFT HDL Optimized/2 -> validOut/1
  dataIn/1 -> FFT HDL Optimized/1
  FFT HDL Optimized/1 -> dataOut/1
  FFT HDL Optimized/3 -> Terminator/1

== system soc_swhw_fpga/FPGA Algorithm Wrapper/Input Adapter/Hamming Window ==
  validIn : Inport
  dataIn : Inport  Port=2
  1-D Lookup Table : Lookup_n-D  NumberOfTableDimensions=1  BreakpointsForDimension1="[0 : frameSize  - 1]"  BreakpointsForDimension1FirstPoint=0  IndexSearchMethod=Evenly spaced points  Table=0.54 - (0.46 * cos((2 * pi * (0 : frameSize -1)) / (frameSize - 1)))  TableDataTypeStr=fixdt(0,quantizationBits,quantizationBits)  InterpMethod=Flat  RemoveProtectionInput=on  InternalRulePriority=Speed  OutDataTypeStr=fixdt(0,quantizationBits,quantizationBits)  RndMeth=Zero
  Constant : Constant  OutDataTypeStr=boolean  SampleTime=-1
  Enabled Counter : Subsystem  TreatAsAtomicUnit=on  mask(Counter){maxCount=frameSize, sampleTime=-1}
      mask prompts: maxCount "Maximum count:"; sampleTime "Sample Time:"
  Product : Product  OutDataTypeStr=fixdt(1, quantizationBits, 0)  RndMeth=Zero  LockScale=on
  Subtract : Sum  Inputs=+-  RndMeth=Simplest
  validOut : Outport  InitialOutput=0
  dataOut : Outport  Port=2  InitialOutput=0
  wires:
  1-D Lookup Table/1 -> Product/1
  Enabled Counter/1(count) -> Subtract/1
  Constant/1 -> Subtract/2
  dataIn/1 -> Product/2
  Subtract/1 -> 1-D Lookup Table/1
  Product/1 -> dataOut/1
  validIn/1 -> validOut/1, Enabled Counter/1(en)

== system soc_swhw_fpga/FPGA Algorithm Wrapper/Input Adapter/Quantize ==
  note: new_value = (old_value - old_bottom) / (old_top - old_bottom) * (new_top - new_bottom) + new_bottom
  validIn : Inport
  dataIn : Inport  Port=2
  Constant : Constant  Value=2 ^ (quantizationBits - 1) - 1  OutDataTypeStr=fixdt(1, quantizationBits, 0)  SampleTime=-1
  Product : Product  OutDataTypeStr=fixdt(1,quantizationBits,0)  RndMeth=Zero
  validOut : Outport  InitialOutput=0
  dataOut : Outport  Port=2  InitialOutput=0
  wires:
  Constant/1 -> Product/2
  validIn/1 -> validOut/1
  Product/1 -> dataOut/1
  dataIn/1 -> Product/1

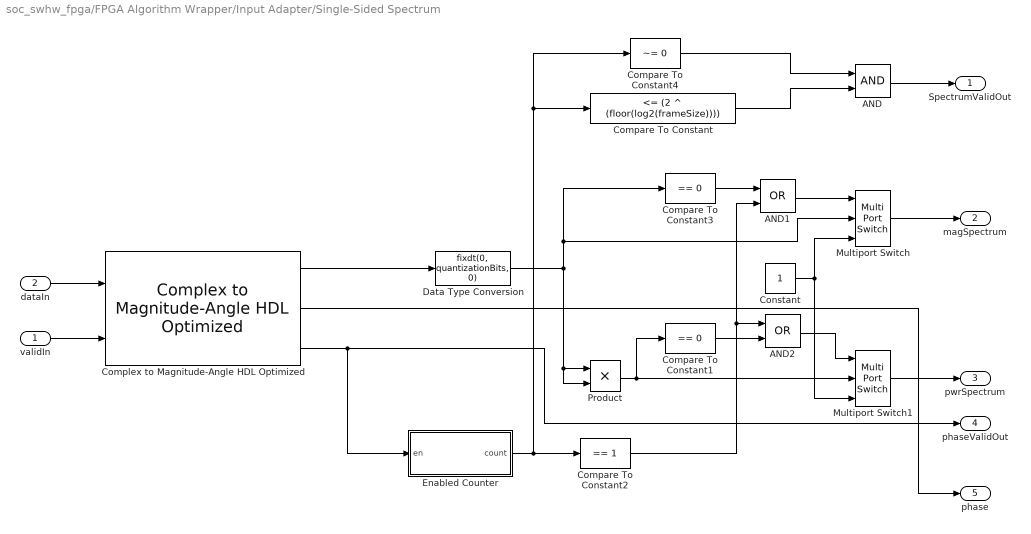
== system soc_swhw_fpga/FPGA Algorithm Wrapper/Input Adapter/Single-Sided Spectrum ==
  validIn : Inport
  dataIn : Inport  Port=2
  AND : Logic  AllPortsSameDT=off  OutDataTypeStr=boolean
  AND1 : Logic  Operator=OR  AllPortsSameDT=off  OutDataTypeStr=boolean
  AND2 : Logic  Operator=OR  AllPortsSameDT=off  OutDataTypeStr=boolean
  Compare To Constant : simulink/Logic and Bit Operations/Compare To Constant  relop=<=  const=(2 ^ (floor(log2(frameSize))))  OutDataTypeStr=boolean
  Compare To Constant1 : simulink/Logic and Bit Operations/Compare To Constant  relop===  const=0  OutDataTypeStr=boolean
  Compare To Constant2 : simulink/Logic and Bit Operations/Compare To Constant  relop===  const=1  OutDataTypeStr=boolean
  Compare To Constant3 : simulink/Logic and Bit Operations/Compare To Constant  relop===  const=0  OutDataTypeStr=boolean
  Compare To Constant4 : simulink/Logic and Bit Operations/Compare To Constant  relop=~=  const=0  OutDataTypeStr=boolean
  Complex to Magnitude-Angle HDL Optimized : dsphdlmathfun/Complex to Magnitude-Angle HDL Optimized  NumIterationsSource=Auto  NumIterations=10  OutputFormat=Magnitude and angle  AngleFormat=Radians  ScaleOutput=on  SimulateUsing=Code generation
      settings: SourceProductBaseCode=DS
  Constant : Constant  OutDataTypeStr=fixdt(0, 1, 0)  SampleTime=-1
  Data Type Conversion : DataTypeConversion  OutDataTypeStr=fixdt(0, quantizationBits, 0)  RndMeth=Simplest
  Enabled Counter : Subsystem  TreatAsAtomicUnit=on  mask(Counter){maxCount=2 ^ (floor(log2(frameSize)) + 1), sampleTime=-1}
      mask prompts: maxCount "Maximum count:"; sampleTime "Sample Time:"
  Multiport Switch : MultiPortSwitch  DataPortOrder=Zero-based contiguous  Inputs=2  zeroidx=on  RndMeth=Simplest
  Multiport Switch1 : MultiPortSwitch  DataPortOrder=Zero-based contiguous  Inputs=2  zeroidx=on  RndMeth=Simplest
  Product : Product
  SpectrumValidOut : Outport
  magSpectrum : Outport  Port=2
  pwrSpectrum : Outport  Port=3
  phaseValidOut : Outport  Port=4
  phase : Outport  Port=5
  wires:
  dataIn/1 -> Complex to Magnitude-Angle HDL Optimized/1
  Compare To Constant2/1 -> AND1/2, AND2/1
  Compare To Constant1/1 -> AND2/2
  Multiport Switch1/1 -> pwrSpectrum/1
  Compare To Constant3/1 -> AND1/1
  Complex to Magnitude-Angle HDL Optimized/1 -> Data Type Conversion/1
  Constant/1 -> Multiport Switch1/3, Multiport Switch/3
  validIn/1 -> Complex to Magnitude-Angle HDL Optimized/2
  Complex to Magnitude-Angle HDL Optimized/3 -> phaseValidOut/1, Enabled Counter/1(en)
  Product/1 -> Compare To Constant1/1, Multiport Switch1/2
  Complex to Magnitude-Angle HDL Optimized/2 -> phase/1
  Multiport Switch/1 -> magSpectrum/1
  Enabled Counter/1(count) -> Compare To Constant4/1, Compare To Constant/1, Compare To Constant2/1
  Compare To Constant/1 -> AND/2
  Compare To Constant4/1 -> AND/1
  AND2/1 -> Multiport Switch1/1
  AND1/1 -> Multiport Switch/1
  AND/1 -> SpectrumValidOut/1
  Data Type Conversion/1 -> Product/2, Product/1, Compare To Constant3/1, Multiport Switch/2

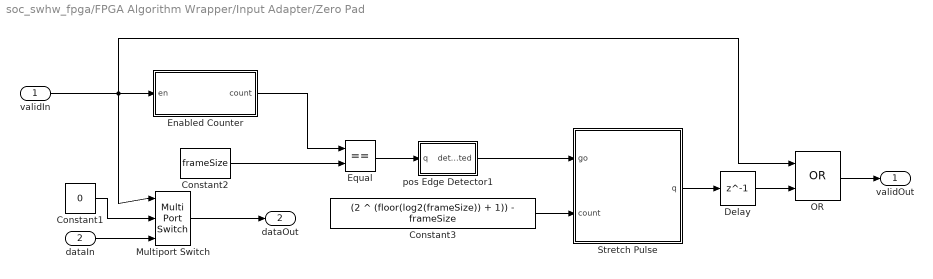
== system soc_swhw_fpga/FPGA Algorithm Wrapper/Input Adapter/Zero Pad ==
  validIn : Inport
  dataIn : Inport  Port=2
  Constant1 : Constant  Value=0  OutDataTypeStr=fixdt(0, 1, 0)  SampleTime=-1
  Constant2 : Constant  Value=frameSize  OutDataTypeStr=fixdt(0, floor(log2(frameSize)) + 1, 0)  SampleTime=-1
  Constant3 : Constant  Value=(2 ^ (floor(log2(frameSize)) + 1)) - frameSize  OutDataTypeStr=fixdt(0, floor(log2((2 ^ (floor(log2(frameSize)) + 1)) - frameSize)) + 1, 0)  SampleTime=-1
  Delay : Delay  DelayLength=1
  Enabled Counter : Subsystem  TreatAsAtomicUnit=on  mask(Counter){maxCount=frameSize, sampleTime=-1}
      mask prompts: maxCount "Maximum count:"; sampleTime "Sample Time:"
  Equal : RelationalOperator  Operator===  OutDataTypeStr=boolean  RndMeth=Simplest
  Multiport Switch : MultiPortSwitch  DataPortOrder=Zero-based contiguous  Inputs=2  zeroidx=on
  OR : Logic  Operator=OR  AllPortsSameDT=off  OutDataTypeStr=boolean
  Stretch Pulse : Subsystem
  pos Edge Detector1 : Subsystem
  validOut : Outport
  dataOut : Outport  Port=2
  wires:
  dataIn/1 -> Multiport Switch/3
  Delay/1 -> OR/2
  Enabled Counter/1(count) -> Equal/1
  Constant2/1 -> Equal/2
  Multiport Switch/1 -> dataOut/1
  Constant1/1 -> Multiport Switch/2
  Equal/1 -> pos Edge Detector1/1(q)
  OR/1 -> validOut/1
  Constant3/1 -> Stretch Pulse/2(count)
  Stretch Pulse/1(q) -> Delay/1
  pos Edge Detector1/1(detected) -> Stretch Pulse/1(go)
  validIn/1 -> OR/1, Multiport Switch/1, Enabled Counter/1(en)

== system soc_swhw_fpga/FPGA Algorithm Wrapper/Output Adapter/De-Quantize ==
  note: new_value = (old_value - old_bottom) / (old_top - old_bottom) * (new_top - new_bottom) + new_bottom
  validIn : Inport
  dataIn : Inport  Port=2
  Constant : Constant  Value=1/ (2 ^ (quantizationBits - 1) - 1)  OutDataTypeStr=fixdt(0,quantizationBits,quantizationBits)  SampleTime=-1
  Product : Product  OutDataTypeStr=fixdt(1,32,30)  RndMeth=Zero
  validOut : Outport  InitialOutput=0
  dataOut : Outport  Port=2  InitialOutput=0
  wires:
  Constant/1 -> Product/2
  dataIn/1 -> Product/1
  validIn/1 -> validOut/1
  Product/1 -> dataOut/1

== system soc_swhw_fpga/FPGA Algorithm Wrapper/Output Adapter/IFFT ==
  validIn : Inport
  dataIn : Inport  Port=2
  Complex to Real-Imag : ComplexToRealImag
  Extract Bits : simulink/Logic and Bit Operations/Extract Bits  bitsToExtract=Range ending with least significant bit  numBits=quantizationBits + 1  bitIdxRange=[0 7]  outScalingMode=Preserve fixed-point scaling
  IFFT HDL Optimized : dsphdlxfrm/IFFT HDL Optimized  FFTLength=(2 ^ (floor(log2(frameSize)) + 1))  Architecture=Burst Radix 2  ComplexMultiplication=Use 3 multipliers and 5 adders  BitReversedOutput=off  BitReversedInput=off  Normalize=off  SimulateUsing=Code generation  RoundingMethod=Zero  ResetInputPort=off  StartOutputPort=off  EndOutputPort=off
      settings: SourceProductBaseCode=DS
  Terminator : Terminator
  Terminator1 : Terminator
  validOut : Outport
  dataOut : Outport  Port=2
  wires:
  validIn/1 -> IFFT HDL Optimized/2
  IFFT HDL Optimized/2 -> validOut/1
  dataIn/1 -> IFFT HDL Optimized/1
  IFFT HDL Optimized/1 -> Complex to Real-Imag/1
  Complex to Real-Imag/2 -> Terminator/1
  Complex to Real-Imag/1 -> Extract Bits/1
  Extract Bits/1 -> dataOut/1
  IFFT HDL Optimized/3 -> Terminator1/1

== system soc_swhw_fpga/FPGA Algorithm Wrapper/Output Adapter/Magnitude and Phase to Complex ==
  magnitudeValidIn : Inport
  magnitudeIn : Inport  Port=2
  phaseValidIn : Inport  Port=3
  phaseIn : Inport  Port=4
  AND : Logic  Operator=NOR  AllPortsSameDT=off  OutDataTypeStr=boolean
  Delay : Delay  DelayLength=1
  HDL FIFO : hdlsllib/HDL RAMs/HDL FIFO  fifo_size=2^(floor(log2(frameSize)) + 1)  mode=Classic  ratio=1  push_msg=Warning  pop_msg=Warning  show_empty=on  show_full=off  show_num=off  LabelModeActiveChoice_Mode=Classic
      settings: SourceProductBaseCode=SL
  HDL FIFO1 : hdlsllib/HDL RAMs/HDL FIFO  fifo_size=2^(floor(log2(frameSize)) + 1)  mode=Classic  ratio=1  push_msg=Warning  pop_msg=Warning  show_empty=on  show_full=off  show_num=off  LabelModeActiveChoice_Mode=Classic
      settings: SourceProductBaseCode=SL
  Product : Product  OutDataTypeStr=fixdt(1, quantizationBits, 0)  RndMeth=Convergent
  Trigonometric Function1 : Trigonometry  Operator=cos + jsin  ApproximationMethod=CORDIC  NumberOfIterations=quantizationBits
  validOut : Outport
  dataOut : Outport  Port=2
  wires:
  HDL FIFO1/1 -> Trigonometric Function1/1
  magnitudeValidIn/1 -> HDL FIFO/2
  magnitudeIn/1 -> HDL FIFO/1
  phaseIn/1 -> HDL FIFO1/1
  phaseValidIn/1 -> HDL FIFO1/2
  Delay/1 -> validOut/1
  Product/1 -> dataOut/1
  AND/1 -> Delay/1, HDL FIFO/3, HDL FIFO1/3
  HDL FIFO1/2 -> AND/2
  HDL FIFO/2 -> AND/1
  Trigonometric Function1/1 -> Product/2
  HDL FIFO/1 -> Product/1

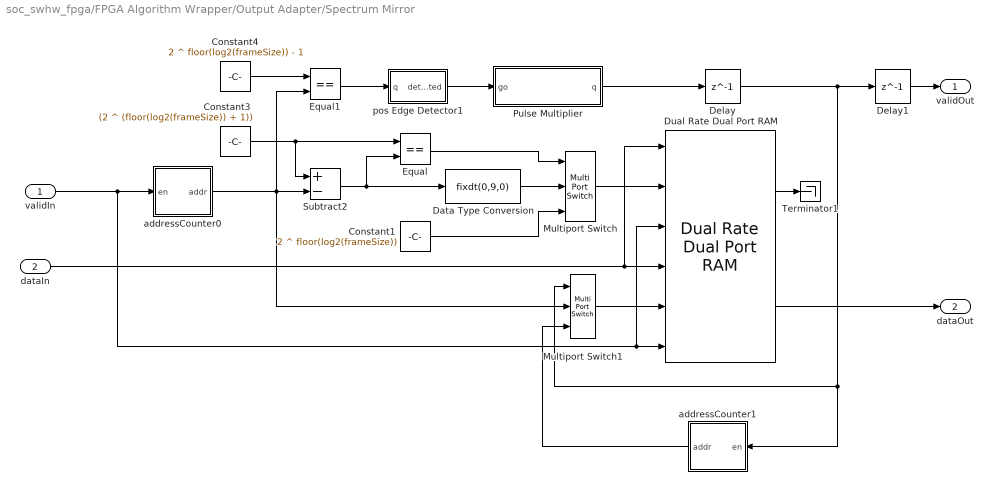
== system soc_swhw_fpga/FPGA Algorithm Wrapper/Output Adapter/Spectrum Mirror ==
  validIn : Inport
  dataIn : Inport  Port=2
  Constant1 : Constant  Value=2 ^ floor(log2(frameSize))  OutDataTypeStr=ufix(floor(log2(frameSize) + 1))  SampleTime=sampleTime
  Constant3 : Constant  Value=(2 ^ (floor(log2(frameSize)) + 1))  OutDataTypeStr=ufix(ceil(log2(frameSize)) + 1)  SampleTime=sampleTime
  Constant4 : Constant  Value=2 ^ floor(log2(frameSize)) - 1  OutDataTypeStr=ufix(floor(log2(frameSize)))  SampleTime=sampleTime
  Data Type Conversion : DataTypeConversion  OutDataTypeStr=fixdt(0,9,0)
  Delay : Delay  DelayLength=1
  Delay1 : Delay  DelayLength=1
  Dual Rate Dual Port RAM : hdlsllib/HDL RAMs/Dual Rate Dual Port RAM  ram_size=floor(log2(frameSize)) + 1
      settings: SourceProductBaseCode=SL
  Equal : RelationalOperator  Operator===  OutDataTypeStr=boolean  RndMeth=Simplest
  Equal1 : RelationalOperator  Operator===  OutDataTypeStr=boolean  RndMeth=Simplest
  Multiport Switch : MultiPortSwitch  DataPortOrder=Zero-based contiguous  Inputs=2  zeroidx=on  RndMeth=Simplest
  Multiport Switch1 : MultiPortSwitch  DataPortOrder=Zero-based contiguous  Inputs=2  zeroidx=on  RndMeth=Simplest
  Pulse Multiplier : Subsystem  mask{N=floor(log2(frameSize)) + 1}
      mask DialogControl Control2 Prompt: Stretches a single-cycle pulse on its input into a 2^N-cycle pulse on its output.The block ignores any input pulse that arrives within 2^N cycles of the previous one.
      mask DialogControl Control3 Prompt: If the PulseMultiplier block receives a second 1 on its input while it is producing an existing stream, its behavior is undefined.
      mask DialogControl Control4 Prompt: Note: this behaviour is different from the original definition of this component.
      mask DialogControl N_text Prompt: N, where one input pulse produces a train of 2^N output pulses.
      mask Display:
      | length = 2 ^str2num(get_param(gcb, 'N'));
      | disp(['Pulse Length:  ' num2str(length)]);
  Subtract2 : Sum  Inputs=+-  RndMeth=Simplest
  Terminator1 : Terminator
  addressCounter0 : Subsystem
  addressCounter1 : Subsystem
  pos Edge Detector1 : Subsystem
  validOut : Outport
  dataOut : Outport  Port=2
  wires:
  validIn/1 -> Dual Rate Dual Port RAM/3, Dual Rate Dual Port RAM/6, addressCounter0/1(en)
  dataIn/1 -> Dual Rate Dual Port RAM/1, Dual Rate Dual Port RAM/4
  Dual Rate Dual Port RAM/2 -> dataOut/1
  Dual Rate Dual Port RAM/1 -> Terminator1/1
  Multiport Switch/1 -> Dual Rate Dual Port RAM/2
  Equal/1 -> Multiport Switch/1
  Subtract2/1 -> Data Type Conversion/1, Equal/2
  Constant1/1 -> Multiport Switch/3
  Multiport Switch1/1 -> Dual Rate Dual Port RAM/5
  addressCounter1/1(addr) -> Multiport Switch1/3
  addressCounter0/1(addr) -> Multiport Switch1/2, Equal1/2, Subtract2/2
  Constant3/1 -> Subtract2/1, Equal/1
  Constant4/1 -> Equal1/1
  Equal1/1 -> pos Edge Detector1/1(q)
  pos Edge Detector1/1(detected) -> Pulse Multiplier/1(go)
  Pulse Multiplier/1(q) -> Delay/1
  Delay/1 -> Delay1/1, Multiport Switch1/1, addressCounter1/1(en)
  Data Type Conversion/1 -> Multiport Switch/2
  Delay1/1 -> validOut/1
